simulink model "OuterLoopController"  (R2014b)
settings: Solver=ode45  StartTime=0.0  StopTime=10.0  RelTol=1e-3
values from neighbouring files (symbols this model uses):
  K_0 = 100*eye(N)    [OpenKinematicChainExample.m]
  K_1 = 50*eye(N)    [OpenKinematicChainExample.m]
settings Model: Creator=tchoopojcharoen  LastModifiedBy=tchoopojcharoen

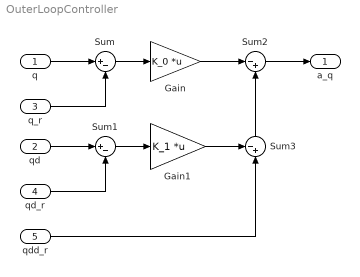
== system OuterLoopController ==
  q : Inport
  qd : Inport  Port=2
  q_r : Inport  Port=3
  qd_r : Inport  Port=4
  qdd_r : Inport  Port=5
  Gain : Gain  Gain=K_0  Multiplication=Matrix(K*u)
  Gain1 : Gain  Gain=K_1  Multiplication=Matrix(K*u)
  Sum : Sum  Inputs=|+-
  Sum1 : Sum  Inputs=|+-
  Sum2 : Sum  Inputs=|-+
  Sum3 : Sum  Inputs=-+|
  a_q : Outport
  wires:
  q/1 -> Sum/1
  q_r/1 -> Sum/2
  qd/1 -> Sum1/1
  qd_r/1 -> Sum1/2
  Sum/1 -> Gain/1
  Sum1/1 -> Gain1/1
  Gain/1 -> Sum2/1
  Gain1/1 -> Sum3/1
  Sum3/1 -> Sum2/2
  qdd_r/1 -> Sum3/2
  Sum2/1 -> a_q/1
